simulink model "SwitchingPreisach"  (R2017b)
settings: Solver=FixedStepAuto  StartTime=0.0  StopTime=simTotalTime  FixedStep=0.05  MaxStep=0.1  MinStep=0.01  RelTol=1e-3
undefined symbols (not defined in the file): GA, GB, GC, GD, gridArea, gridDen, gridLength, Gx0, hysteronMax, hysteronMin, initialInput, initialRelays, inputAmp, inputFactor, inputMax, inputMin, offset, outputAmp, outputFactor, outputMax, outputMin, weightFunc, xyGrid
libraries: simulink x2
settings Model: Creator=Marco  LastModifiedBy=M. Vasquez Beltran

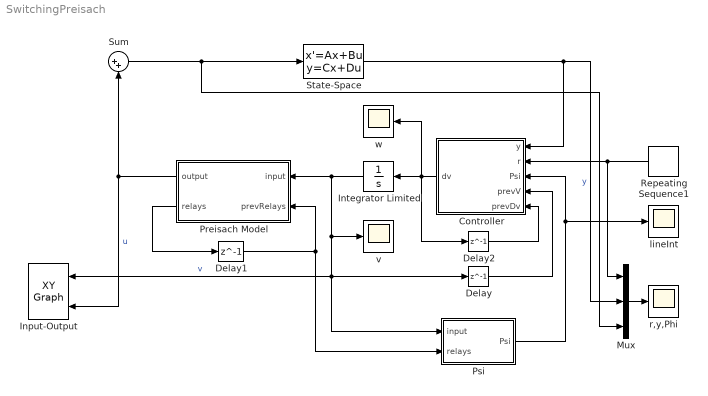
== system SwitchingPreisach ==
  Controller : MATLAB Function  TreatAsAtomicUnit=on
  Delay : Delay  DelayLength=1
  Delay1 : Delay  DelayLength=1  InitialCondition=initialRelays
  Delay2 : Delay  DelayLength=1
  Input-Output : simulink/Sinks/XY Graph  xmin=inputMin - inputAmp*inputFactor  xmax=inputMax + inputAmp*inputFactor  ymin=outputMin - outputAmp*outputFactor  ymax=outputMax + outputAmp*outputFactor  st=-1
  Integrator Limited : Integrator  InitialCondition=initialInput  UpperSaturationLimit=inputMax*0.99  LowerSaturationLimit=inputMin*0.99
  Mux : Mux  Inputs=3
  Preisach Model : MATLAB Function  TreatAsAtomicUnit=on
  Psi : MATLAB Function  TreatAsAtomicUnit=on
  Repeating Sequence1 : simulink/Sources/Repeating Sequence  rep_seq_t=sequenceTime  rep_seq_y=sequenceVal
  State-Space : StateSpace  A=GA  B=GB  C=GC  D=GD  InitialCondition=Gx0
  Sum : Sum  Inputs=|++
  lineInt : Scope
  r,y,Phi : Scope
  v : Scope
  w : Scope
  wires:
  Preisach Model/2(relays) -> Delay1/1
  Delay1/1 -> Preisach Model/2(prevRelays), Psi/2(relays)
  Sum/1 -> Mux/3, State-Space/1
  Preisach Model/1(output) -> Input-Output/2, Sum/2  "u"
  State-Space/1 -> Controller/1(y), Mux/2  "y"
  Integrator Limited/1 -> Psi/1(input), Input-Output/1, Delay/1, v/1, Preisach Model/1(input)  "v"
  Repeating Sequence1/1 -> Mux/1, Controller/2(r)
  Controller/1(dv) -> Delay2/1, Integrator Limited/1, w/1
  Mux/1 -> r,y,Phi/1
  Psi/1(Psi) -> lineInt/1, Controller/3(Psi)
  Delay2/1 -> Controller/5(prevDv)
  Delay/1 -> Controller/4(prevV)

== matlab function SwitchingPreisach/Preisach Model ==
  data: input input; prevRelays input; output output; weightFunc parameter; relays output; offset parameter; hysteronMin parameter; hysteronMax parameter; gridDen parameter; xyGrid parameter; gridLength parameter; gridArea parameter
function [output, relays] = fcn(input, prevRelays, ...
    weightFunc, offset, hysteronMin, hysteronMax, gridDen, xyGrid, gridLength, gridArea)

    relays = prevRelays;
    if( xyGrid(end) <= input )
        relays(:,:) = hysteronMax*fliplr(triu(ones(gridDen, gridDen)));
    elseif( input < xyGrid(1) )
        relays(:,:) = hysteronMin*fliplr(triu(ones(gridDen, gridDen)));
    else
        idx0 = 1;
        while( idx0 <= gridDen-1 )
            if( xyGrid(idx0) <= input && input < xyGrid(idx0+1) )
                col = idx0;
                row = gridDen-idx0+1;

                relays(row:end, 1:col) = hysteronMax*fliplr(triu(ones(col, col)));
                relays(1:row-1, col+1:end) = hysteronMin*fliplr(triu(ones(row-1, row-1)));
                break;
            end
            idx0 = idx0 + 1;
        end
    end
    output = sum(sum(relays(:,:).*weightFunc(:,:)))*gridArea + offset;

== matlab function SwitchingPreisach/Psi ==
  settings: updateMethod=DISCRETE
  data: input input; relays input; weightFunc parameter; hysteronMin parameter; hysteronMax parameter; offset parameter; gridDen parameter; Psi output; xyGrid parameter; gridLength parameter
function Psi = fcn(input, relays,...
     weightFunc, hysteronMin, hysteronMax, offset, gridDen, xyGrid, gridLength)

Psi = [0; 0] + [(rand()-0.5); (rand()-0.5)]/10;
if( xyGrid(end) <= input )
    return;
elseif( input < xyGrid(1) )
    return;
else
    idx0 = 1;
    while( idx0 <= gridDen-1 )
        if( xyGrid(idx0) <= input && input < xyGrid(idx0+1) )
            col = idx0;
            row = gridDen-idx0+1;
            
            for var=col:-1:1
                if( relays(row-1,var)==hysteronMin )
                    Psi(1) = Psi(1) + gridLength*weightFunc(row-1,var);
                end
            end
            
            for var=row:-1:1
                if( relays(var,col)==hysteronMax )
                    Psi(2) = Psi(2) + gridLength*weightFunc(var,col);
                end
            end
            
            break;
        end
        idx0 = idx0 + 1;
    end
end
Psi = 2*Psi;

end

== matlab function SwitchingPreisach/Controller ==
  settings: updateMethod=DISCRETE
  data: y input; r input; Psi input; prevV input; prevDv input; dv output; inputMin parameter; inputMax parameter
function dv = fcn(y, r, Psi, prevV, prevDv, inputMin, inputMax)
    
    %%%%%%%%%%%%%%%%%%%%%%%%%%%%%%%%%%%%%%%%%%%%%%%%%%%%%%%%%%%%%%%%%%%%%%%
    % Params
    %%%%%%%%%%%%%%%%%%%%%%%%%%%%%%%%%%%%%%%%%%%%%%%%%%%%%%%%%%%%%%%%%%%%%%%
    gain = 0.5;
    threshold = 0.15;
    error = y-r;
    
    %%%%%%%%%%%%%%%%%%%%%%%%%%%%%%%%%%%%%%%%%%%%%%%%%%%%%%%%%%%%%%%%%%%%%%%
    % Selecting the last value of nonliearity psi
    %%%%%%%%%%%%%%%%%%%%%%%%%%%%%%%%%%%%%%%%%%%%%%%%%%%%%%%%%%%%%%%%%%%%%%%
    if(sign(prevDv)>0)
        prevPsi=Psi(1);
    elseif(sign(prevDv)<0)
        prevPsi=Psi(2);
    else
        prevPsi=0;
    end
    
    %%%%%%%%%%%%%%%%%%%%%%%%%%%%%%%%%%%%%%%%%%%%%%%%%%%%%%%%%%%%%%%%%%%%%%%
    % Control logic
    %%%%%%%%%%%%%%%%%%%%%%%%%%%%%%%%%%%%%%%%%%%%%%%%%%%%%%%%%%%%%%%%%%%%%%% 
    if( prevPsi~=0 )
        lambda = sign(prevPsi)/max([abs(prevPsi), threshold]);
    else
        lambda = 1/max([abs(prevPsi), threshold]);
    end
    dv = -gain*error*lambda;
    
end
